simulink model "PRDPLL"  (R2017b)
settings: Solver=ode45  StartTime=0.0  StopTime=1e-3  RelTol=1e-3  EnableMultiTasking=on
values from neighbouring files (symbols this model uses):
  ki = 1e-6    (= 1e-06)    [PRDPLL_init.m]
  kp = 1e-3    (= 0.001)    [PRDPLL_init.m]
libraries: simulink x9
settings Model: Creator=Tony  LastModifiedBy=Tony
settings DataIOCC: LimitDataPoints=on  SaveFormat=Array
settings OptimizationCC: LifeSpan=inf
settings DebuggingCC: SolverPrmCheckMsg=warning  SFUnexpectedBacktrackingDiag=warning  SFNoUnconditionalDefaultTransitionDiag=warning  SFExecutionAtInitializationDiag=none
settings HardwareCC: ProdBitPerPointer=32  ProdBitPerSizeT=32  ProdBitPerPtrDiffT=32  ProdLargestAtomicFloat=None  ProdIntDivRoundTo=Undefined  ProdEndianess=Unspecified  ProdWordSize=32  ProdHWDeviceType=32-bit Generic
settings ModelReferenceCC: PropagateSignalLabelsOutOfModel=off
settings CodeAppCC: StateflowObjectComments=on
settings GRTTargetCC: TargetLangStandard=C89/C90 (ANSI)  GeneratePreprocessorConditionals=Disable all
settings ConfigComp: CovMetricSettings=dw  CovHtmlReporting=on  CovSaveCumulativeToWorkspaceVar=on  CovSaveSingleToWorkspaceVar=on  CovExternalEMLEnable=off  CovSFcnEnable=off

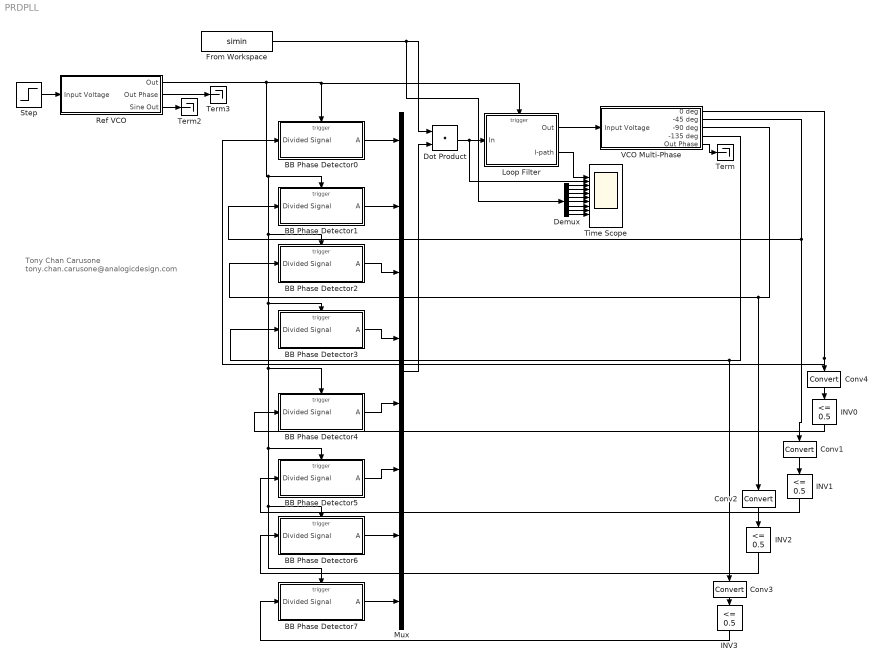
== system PRDPLL ==
  note: Tony Chan Carusone
      | tony.chan.carusone@analogicdesign.com
  BB Phase Detector0 : Subsystem
  BB Phase Detector1 : Subsystem
  BB Phase Detector2 : Subsystem
  BB Phase Detector3 : Subsystem
  BB Phase Detector4 : Subsystem
  BB Phase Detector5 : Subsystem
  BB Phase Detector6 : Subsystem
  BB Phase Detector7 : Subsystem
  Conv{1..4} (4 alike) : DataTypeConversion
  Demux : Demux  Outputs=8
  Dot Product : DotProduct  InputSameDT=on  OutDataTypeStr=Inherit: Inherit via internal rule
  From Workspace : FromWorkspace  VariableName=simin  SampleTime=1/frotate/8  Interpolate=off  OutputAfterFinalValue=Cyclic repetition
  INV{0..3} (4 alike) : simulink/Logic and Bit Operations/Compare To Constant  relop=<=  const=0.5  OutDataTypeStr=uint8
  Loop Filter : Subsystem
  Mux : Mux  Inputs=8
  Ref VCO : Subsystem  mask{Kvco=0, Ac=1, fo=1000e6}
      mask prompts: fo "Default Frequency (fo)"
  Step : Step  Time=0  SampleTime=0
  Term : Terminator
  Term2 : Terminator
  Term3 : Terminator
  Time Scope : Scope  NumInputPorts=10
  VCO Multi-Phase : Subsystem  mask{Kvco=1e9*2*pi, fo=1000e6}
      mask prompts: fo "Default Frequency (fo)"
  wires:
  Loop Filter/1(Out) -> VCO Multi-Phase/1(Input Voltage)
  Ref VCO/1(Out) -> BB Phase Detector5/Trigger, BB Phase Detector7/Trigger, BB Phase Detector6/Trigger, BB Phase Detector4/Trigger, BB Phase Detector3/Trigger, BB Phase Detector2/Trigger, BB Phase Detector1/Trigger, Loop Filter/Trigger, BB Phase Detector0/Trigger
  Step/1 -> Ref VCO/1(Input Voltage)
  VCO Multi-Phase/5(Out Phase) -> Term/1
  Ref VCO/3(Sine Out) -> Term2/1
  Ref VCO/2(Out Phase) -> Term3/1
  Loop Filter/2(I-path) -> Time Scope/1
  VCO Multi-Phase/1(0 deg) -> BB Phase Detector0/1(Divided Signal), Conv4/1
  VCO Multi-Phase/2(-45 deg) -> BB Phase Detector1/1(Divided Signal), Conv1/1
  VCO Multi-Phase/3(-90 deg) -> BB Phase Detector2/1(Divided Signal), Conv2/1
  VCO Multi-Phase/4(-135 deg) -> BB Phase Detector3/1(Divided Signal), Conv3/1
  INV0/1 -> BB Phase Detector4/1(Divided Signal)
  INV1/1 -> BB Phase Detector5/1(Divided Signal)
  INV2/1 -> BB Phase Detector6/1(Divided Signal)
  INV3/1 -> BB Phase Detector7/1(Divided Signal)
  BB Phase Detector0/1(A) -> Mux/1
  BB Phase Detector1/1(A) -> Mux/2
  BB Phase Detector6/1(A) -> Mux/7
  BB Phase Detector7/1(A) -> Mux/8
  BB Phase Detector5/1(A) -> Mux/6
  BB Phase Detector4/1(A) -> Mux/5
  BB Phase Detector3/1(A) -> Mux/4
  BB Phase Detector2/1(A) -> Mux/3
  Dot Product/1 -> Time Scope/2, Loop Filter/1(In)
  Mux/1 -> Dot Product/2
  From Workspace/1 -> Demux/1, Dot Product/1
  Demux/1 -> Time Scope/3
  Demux/2 -> Time Scope/4
  Demux/3 -> Time Scope/5
  Demux/4 -> Time Scope/6
  Demux/5 -> Time Scope/7
  Demux/6 -> Time Scope/8
  Demux/7 -> Time Scope/9
  Demux/8 -> Time Scope/10
  Conv3/1 -> INV3/1
  Conv1/1 -> INV1/1
  Conv2/1 -> INV2/1
  Conv4/1 -> INV0/1

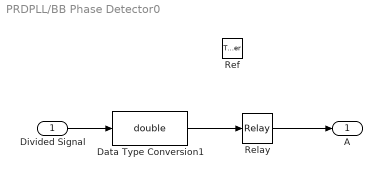
== system PRDPLL/BB Phase Detector0 ==
  Divided Signal : Inport
  Ref : TriggerPort  VariantControl=(inherit)
  Data Type Conversion1 : DataTypeConversion  OutDataTypeStr=double
  Relay : Relay  OffOutputValue=-1
  A : Outport
  wires:
  Relay/1 -> A/1
  Divided Signal/1 -> Data Type Conversion1/1
  Data Type Conversion1/1 -> Relay/1

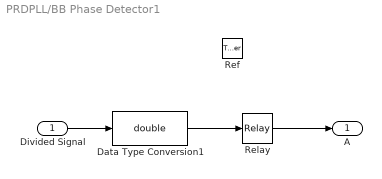
== system PRDPLL/BB Phase Detector1 ==
  Divided Signal : Inport
  Ref : TriggerPort  VariantControl=(inherit)
  Data Type Conversion1 : DataTypeConversion  OutDataTypeStr=double
  Relay : Relay  OffOutputValue=-1
  A : Outport
  wires:
  Data Type Conversion1/1 -> Relay/1
  Divided Signal/1 -> Data Type Conversion1/1
  Relay/1 -> A/1

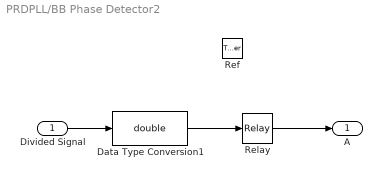
== system PRDPLL/BB Phase Detector2 ==
  Divided Signal : Inport
  Ref : TriggerPort  VariantControl=(inherit)
  Data Type Conversion1 : DataTypeConversion  OutDataTypeStr=double
  Relay : Relay  OffOutputValue=-1
  A : Outport
  wires:
  Relay/1 -> A/1
  Divided Signal/1 -> Data Type Conversion1/1
  Data Type Conversion1/1 -> Relay/1

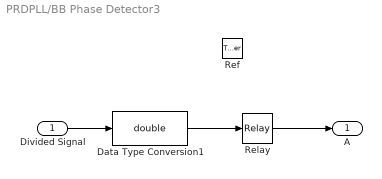
== system PRDPLL/BB Phase Detector3 ==
  Divided Signal : Inport
  Ref : TriggerPort  VariantControl=(inherit)
  Data Type Conversion1 : DataTypeConversion  OutDataTypeStr=double
  Relay : Relay  OffOutputValue=-1
  A : Outport
  wires:
  Data Type Conversion1/1 -> Relay/1
  Divided Signal/1 -> Data Type Conversion1/1
  Relay/1 -> A/1

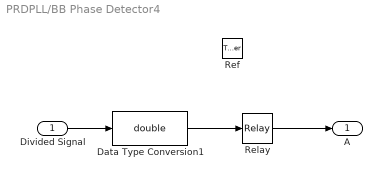
== system PRDPLL/BB Phase Detector4 ==
  Divided Signal : Inport
  Ref : TriggerPort  VariantControl=(inherit)
  Data Type Conversion1 : DataTypeConversion  OutDataTypeStr=double
  Relay : Relay  OffOutputValue=-1
  A : Outport
  wires:
  Data Type Conversion1/1 -> Relay/1
  Divided Signal/1 -> Data Type Conversion1/1
  Relay/1 -> A/1

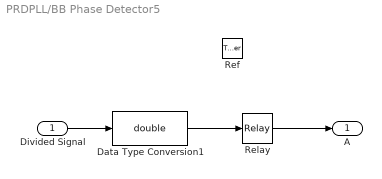
== system PRDPLL/BB Phase Detector5 ==
  Divided Signal : Inport
  Ref : TriggerPort  VariantControl=(inherit)
  Data Type Conversion1 : DataTypeConversion  OutDataTypeStr=double
  Relay : Relay  OffOutputValue=-1
  A : Outport
  wires:
  Relay/1 -> A/1
  Divided Signal/1 -> Data Type Conversion1/1
  Data Type Conversion1/1 -> Relay/1

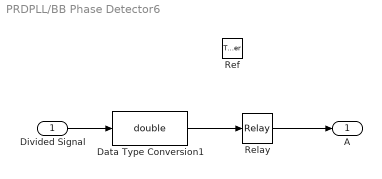
== system PRDPLL/BB Phase Detector6 ==
  Divided Signal : Inport
  Ref : TriggerPort  VariantControl=(inherit)
  Data Type Conversion1 : DataTypeConversion  OutDataTypeStr=double
  Relay : Relay  OffOutputValue=-1
  A : Outport
  wires:
  Data Type Conversion1/1 -> Relay/1
  Divided Signal/1 -> Data Type Conversion1/1
  Relay/1 -> A/1

== system PRDPLL/BB Phase Detector7 ==
  Divided Signal : Inport
  Ref : TriggerPort  VariantControl=(inherit)
  Data Type Conversion1 : DataTypeConversion  OutDataTypeStr=double
  Relay : Relay  OffOutputValue=-1
  A : Outport
  wires:
  Relay/1 -> A/1
  Divided Signal/1 -> Data Type Conversion1/1
  Data Type Conversion1/1 -> Relay/1

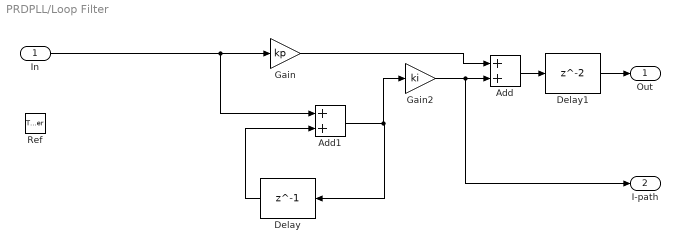
== system PRDPLL/Loop Filter ==
  In : Inport
  Ref : TriggerPort  VariantControl=(inherit)
  Add : Sum
  Add1 : Sum
  Delay : Delay  DelayLength=1  InitialCondition=0  InputProcessing=Inherited
  Delay1 : Delay  InitialCondition=0  InputProcessing=Inherited
  Gain : Gain  Gain=kp
  Gain2 : Gain  Gain=ki
  Out : Outport
  I-path : Outport  Port=2
  wires:
  Delay/1 -> Add1/2
  Gain/1 -> Add/1
  Add1/1 -> Gain2/1, Delay/1
  Add/1 -> Delay1/1
  Delay1/1 -> Out/1
  Gain2/1 -> I-path/1, Add/2
  In/1 -> Add1/1, Gain/1

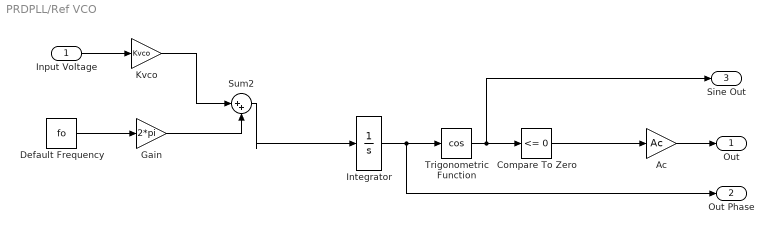
== system PRDPLL/Ref VCO ==
  Input Voltage : Inport
  Ac : Gain  Gain=Ac
  Compare To Zero : simulink/Logic and Bit Operations/Compare To Zero  relop=<=  OutDataTypeStr=uint8
  Default Frequency : Constant  Value=fo
  Gain : Gain  Gain=2*pi
  Integrator : Integrator
  Kvco : Gain  Gain=Kvco
  Sum2 : Sum  Inputs=|++
  Trigonometric Function : Trigonometry  Operator=cos
  Out : Outport
  Out Phase : Outport  Port=2
  Sine Out : Outport  Port=3
  wires:
  Ac/1 -> Out/1
  Compare To Zero/1 -> Ac/1
  Trigonometric Function/1 -> Sine Out/1, Compare To Zero/1
  Default Frequency/1 -> Gain/1
  Input Voltage/1 -> Kvco/1
  Integrator/1 -> Out Phase/1, Trigonometric Function/1
  Sum2/1 -> Integrator/1
  Gain/1 -> Sum2/2
  Kvco/1 -> Sum2/1

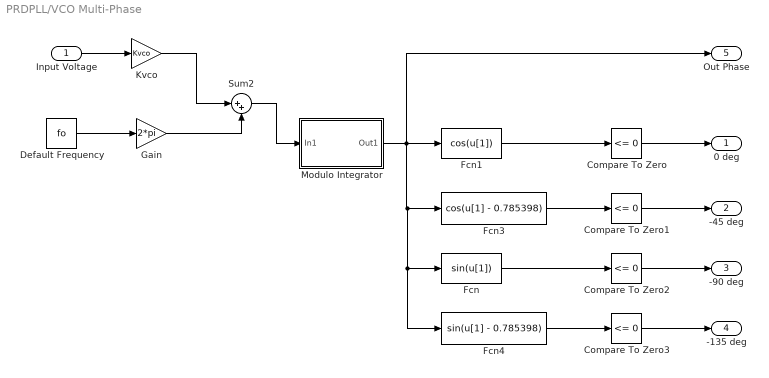
== system PRDPLL/VCO Multi-Phase ==
  Input Voltage : Inport
  Compare To Zero{,1..3} (4 alike) : simulink/Logic and Bit Operations/Compare To Zero  relop=<=  OutDataTypeStr=uint8
  Default Frequency : Constant  Value=fo
  Fcn : Fcn
  Fcn1 : Fcn  Expr=cos(u[1])
  Fcn3 : Fcn  Expr=cos(u[1] - 0.785398)
  Fcn4 : Fcn  Expr=sin(u[1] - 0.785398)
  Gain : Gain  Gain=2*pi
  Kvco : Gain  Gain=Kvco  OutDataTypeStr=Inherit: Inherit via back propagation
  Modulo Integrator : Subsystem
  Sum2 : Sum  Inputs=|++
  0 deg : Outport
  -45 deg : Outport  Port=2
  -90 deg : Outport  Port=3
  -135 deg : Outport  Port=4
  Out Phase : Outport  Port=5
  wires:
  Kvco/1 -> Sum2/1
  Gain/1 -> Sum2/2
  Sum2/1 -> Modulo Integrator/1(In1)
  Modulo Integrator/1(Out1) -> Fcn4/1, Fcn/1, Fcn3/1, Fcn1/1, Out Phase/1
  Input Voltage/1 -> Kvco/1
  Default Frequency/1 -> Gain/1
  Fcn4/1 -> Compare To Zero3/1
  Fcn3/1 -> Compare To Zero1/1
  Fcn1/1 -> Compare To Zero/1
  Fcn/1 -> Compare To Zero2/1
  Compare To Zero/1 -> 0 deg/1
  Compare To Zero1/1 -> -45 deg/1
  Compare To Zero2/1 -> -90 deg/1
  Compare To Zero3/1 -> -135 deg/1

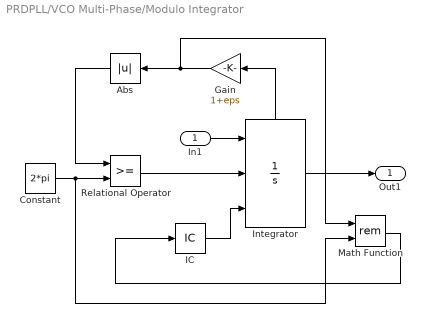
== system PRDPLL/VCO Multi-Phase/Modulo Integrator ==
  In1 : Inport
  Abs : Abs  SaturateOnIntegerOverflow=on
  Constant : Constant  Value=2*pi
  Gain : Gain  Gain=1+eps  SaturateOnIntegerOverflow=on  OutDataTypeStr=Inherit: Same as input  ParamDataTypeStr=Inherit: Same as input
  IC : InitialCondition  Value=0
  Integrator : Integrator  ExternalReset=rising  InitialConditionSource=external  UpperSaturationLimit=1  LowerSaturationLimit=0  ShowStatePort=on
  Math Function : Math  Operator=rem  SaturateOnIntegerOverflow=on
  Relational Operator : RelationalOperator  RndMeth=Nearest  InputSameDT=on
  Out1 : Outport
  wires:
  IC/1 -> Integrator/3
  In1/1 -> Integrator/1
  Integrator/1 -> Out1/1
  Math Function/1 -> IC/1
  Abs/1 -> Relational Operator/1
  Relational Operator/1 -> Integrator/2
  Constant/1 -> Math Function/2, Relational Operator/2
  Integrator/State -> Gain/1
  Gain/1 -> Abs/1, Math Function/1
